simulink model "CommandArbitration"  (R2026a)
settings: Solver=FixedStepDiscrete  StopTime=10  FixedStep=0.01
model workspace (MAT data in the model file):
  P.prio_elrs = 110
  P.prio_joystick = 100
  P.prio_driver_interface = 8
  P.prio_nav = 5
  P.timeout_elrs = 0.5
  P.timeout_joystick = 0.5
  P.timeout_driver_interface = 0.3
  P.timeout_nav = 0.5
  P.prio_motion_lock = 200
  P.timeout_motion_lock = 0.5
  P.motion_lock_rate = 10
  P.motion_lock_gpio_timeout = 1
  P.cmd_vel_timeout = 0.5
  P.diff_drive_update_rate = 50
  P.max_linear_velocity = 0.95
  P.max_linear_acceleration = 2.7
  P.max_angular_velocity = 1.5
  P.max_angular_acceleration = 3.74
  P.dt = 0.01
Description:
  | As-built command arbitration (rover_twist_mux + rover_controller diff_drive limits). Generated by scripts/build_command_arbitration.m.
settings Model: Creator=potlo  LastModifiedBy=potlo
settings DataIOCC: LoadExternalInput=on

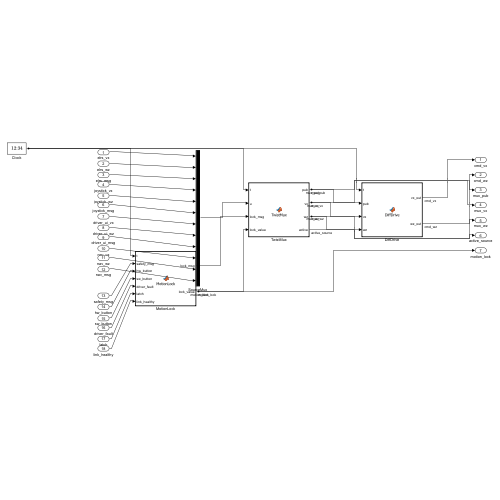
[thumbnail: Simulink's stored preview of the top-level diagram]
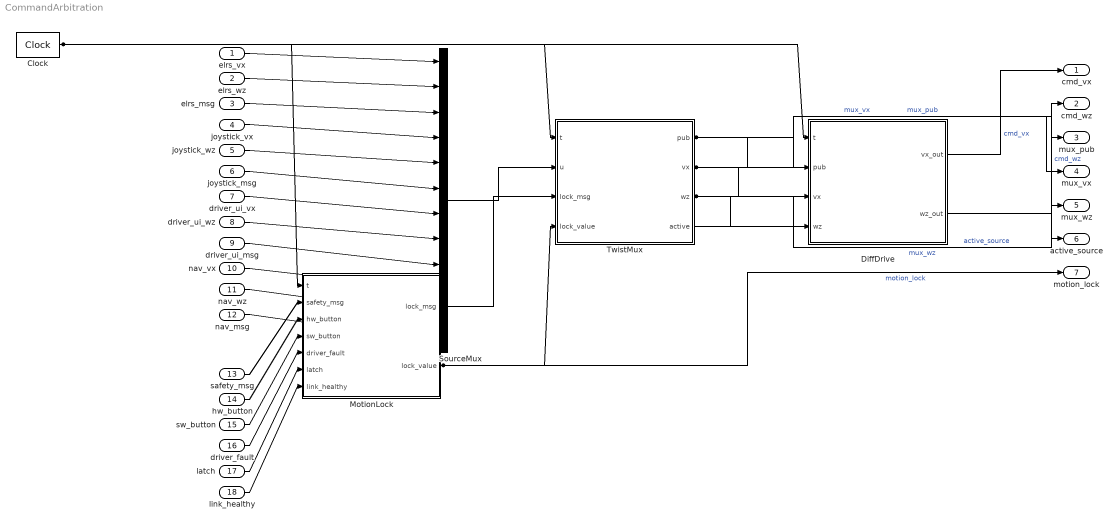
== system CommandArbitration ==
  elrs_vx : Inport  Interpolate=off
  elrs_wz : Inport  Port=2  Interpolate=off
  elrs_msg : Inport  Port=3  Interpolate=off
  joystick_vx : Inport  Port=4  Interpolate=off
  joystick_wz : Inport  Port=5  Interpolate=off
  joystick_msg : Inport  Port=6  Interpolate=off
  driver_ui_vx : Inport  Port=7  Interpolate=off
  driver_ui_wz : Inport  Port=8  Interpolate=off
  driver_ui_msg : Inport  Port=9  Interpolate=off
  nav_vx : Inport  Port=10  Interpolate=off
  nav_wz : Inport  Port=11  Interpolate=off
  nav_msg : Inport  Port=12  Interpolate=off
  safety_msg : Inport  Port=13  Interpolate=off
  hw_button : Inport  Port=14  Interpolate=off
  sw_button : Inport  Port=15  Interpolate=off
  driver_fault : Inport  Port=16  Interpolate=off
  latch : Inport  Port=17  Interpolate=off
  link_healthy : Inport  Port=18  Interpolate=off
  Clock : DigitalClock  SampleTime=0.01
  DiffDrive : MATLAB Function  TreatAsAtomicUnit=on
  MotionLock : MATLAB Function  TreatAsAtomicUnit=on
  SourceMux : Mux  Inputs=12
  TwistMux : MATLAB Function  TreatAsAtomicUnit=on
  cmd_vx : Outport
  cmd_wz : Outport  Port=2
  mux_pub : Outport  Port=3
  mux_vx : Outport  Port=4
  mux_wz : Outport  Port=5
  active_source : Outport  Port=6
  motion_lock : Outport  Port=7
  wires:
  elrs_vx/1 -> SourceMux/1
  elrs_wz/1 -> SourceMux/2
  elrs_msg/1 -> SourceMux/3
  joystick_vx/1 -> SourceMux/4
  joystick_wz/1 -> SourceMux/5
  joystick_msg/1 -> SourceMux/6
  driver_ui_vx/1 -> SourceMux/7
  driver_ui_wz/1 -> SourceMux/8
  driver_ui_msg/1 -> SourceMux/9
  nav_vx/1 -> SourceMux/10
  nav_wz/1 -> SourceMux/11
  nav_msg/1 -> SourceMux/12
  safety_msg/1 -> MotionLock/2(safety_msg)
  hw_button/1 -> MotionLock/3(hw_button)
  sw_button/1 -> MotionLock/4(sw_button)
  driver_fault/1 -> MotionLock/5(driver_fault)
  latch/1 -> MotionLock/6(latch)
  link_healthy/1 -> MotionLock/7(link_healthy)
  Clock/1 -> MotionLock/1(t), TwistMux/1(t), DiffDrive/1(t)
  SourceMux/1 -> TwistMux/2(u)
  MotionLock/1(lock_msg) -> TwistMux/3(lock_msg)
  MotionLock/2(lock_value) -> TwistMux/4(lock_value), motion_lock/1  "motion_lock"
  TwistMux/1(pub) -> DiffDrive/2(pub), mux_pub/1  "mux_pub"
  TwistMux/2(vx) -> DiffDrive/3(vx), mux_vx/1  "mux_vx"
  TwistMux/3(wz) -> DiffDrive/4(wz), mux_wz/1  "mux_wz"
  DiffDrive/1(vx_out) -> cmd_vx/1  "cmd_vx"
  DiffDrive/2(wz_out) -> cmd_wz/1  "cmd_wz"
  TwistMux/4(active) -> active_source/1  "active_source"

== matlab function CommandArbitration/TwistMux ==
  data: t input; u input; pub output; lock_msg input; lock_value input; vx output; wz output; active output; P parameter
function [pub, vx, wz, active] = TwistMux(t, u, lock_msg, lock_value, P)
% u = [vx wz msg] x 4 sources (ELRS, joystick, driver UI, nav).
persistent stamp lock_stamp lock_data
if isempty(stamp), stamp = -inf(1, 4); lock_stamp = -inf; lock_data = 0; end
prio = [P.prio_elrs P.prio_joystick P.prio_driver_interface P.prio_nav];
tout = [P.timeout_elrs P.timeout_joystick P.timeout_driver_interface P.timeout_nav];
if lock_msg > 0.5, lock_stamp = t; lock_data = lock_value; end
locked = (t - lock_stamp) > P.timeout_motion_lock || lock_data > 0.5;
lock_prio = 0;
if locked, lock_prio = P.prio_motion_lock; end
arrived = false(1, 4);
for k = 1:4
    if u(3 * k) > 0.5, stamp(k) = t; arrived(k) = true; end
end
masked = ((t - stamp) > tout) | (prio < lock_prio);
best = 0; bestPrio = -1;
for k = 1:4
    if ~masked(k) && prio(k) > bestPrio, best = k; bestPrio = prio(k); end
end
pub = 0; vx = 0; wz = 0; active = best;
if best > 0 && arrived(best)
    pub = 1; vx = u(3 * best - 2); wz = u(3 * best - 1);
end

== matlab function CommandArbitration/MotionLock ==
  data: t input; lock_msg output; safety_msg input; hw_button input; sw_button input; driver_fault input; latch input; link_healthy input; lock_value output; P parameter
function [lock_msg, lock_value] = MotionLock(t, safety_msg, hw_button, sw_button, driver_fault, latch, link_healthy, P)
% rover_motion_lock_node: publishes motion_lock at motion_lock_rate.
persistent last_rx inhibit next_pub
if isempty(last_rx), last_rx = -inf; inhibit = true; next_pub = 0; end
if safety_msg > 0.5
    last_rx = t;
    inhibit = hw_button > 0.5 || sw_button > 0.5 || driver_fault > 0.5 || latch > 0.5 || link_healthy < 0.5;
end
stale = (t - last_rx) > P.motion_lock_gpio_timeout;
lock_value = double(inhibit || stale);
lock_msg = 0;
if t >= next_pub - 1e-9
    lock_msg = 1;
    next_pub = t + 1 / P.motion_lock_rate;
end

== matlab function CommandArbitration/DiffDrive ==
  data: t input; vx_out output; pub input; vx input; wz input; wz_out output; P parameter
function [vx_out, wz_out] = DiffDrive(t, pub, vx, wz, P)
% diff_drive_controller: runs at diff_drive_update_rate, speed limiter per axis.
persistent last_vx last_wz last_stamp out_vx out_wz next_update
if isempty(last_vx), last_vx = 0; last_wz = 0; last_stamp = -inf; out_vx = 0; out_wz = 0; next_update = 0; end
if pub > 0.5, last_vx = vx; last_wz = wz; last_stamp = t; end
if t >= next_update - 1e-9
    dt = 1 / P.diff_drive_update_rate;
    next_update = t + dt;
    tv = last_vx; tw = last_wz;
    if (t - last_stamp) > P.cmd_vel_timeout, tv = 0; tw = 0; end
    tv = min(max(tv, -P.max_linear_velocity), P.max_linear_velocity);
    tw = min(max(tw, -P.max_angular_velocity), P.max_angular_velocity);
    dv = P.max_linear_acceleration * dt; dw = P.max_angular_acceleration * dt;
    out_vx = out_vx + min(max(tv - out_vx, -dv), dv);
    out_wz = out_wz + min(max(tw - out_wz, -dw), dw);
end
vx_out = out_vx; wz_out = out_wz;
